simulink model "Inverted_Pendulum_on_a_Cart"  (R2018a)
settings: Solver=VariableStepAuto  StartTime=0.0  StopTime=30  RelTol=1e-3
values from neighbouring files (symbols this model uses):
  g = -9.81    [Matlab_Inverted_Pendulum_on_a_Cart.m]
  l = 2    [Matlab_Inverted_Pendulum_on_a_Cart.m]
  M = 5    [Matlab_Inverted_Pendulum_on_a_Cart.m]
  m = 1    [Matlab_Inverted_Pendulum_on_a_Cart.m]
undefined symbols (not defined in the file or in its folder): magnitude
settings Model: Creator=lucas  LastModifiedBy=root
settings DataIOCC: ReturnWorkspaceOutputs=on
settings SFSimCC: SimUseLocalCustomCode=on
settings RTWCC: RTWUseLocalCustomCode=on

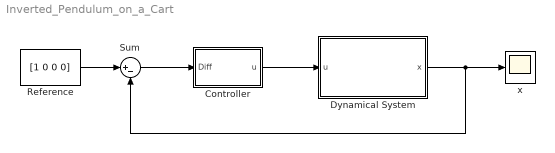
== system Inverted_Pendulum_on_a_Cart ==
  Controller : Subsystem
  Dynamical System : Subsystem
  Reference : Constant  Value=[1 0 0 0]  VectorParams1D=off
  Sum : Sum  Inputs=|+-
  x : Scope
  wires:
  Reference/1 -> Sum/1
  Sum/1 -> Controller/1(Diff)
  Controller/1(u) -> Dynamical System/1(u)
  Dynamical System/1(x) -> x/1, Sum/2

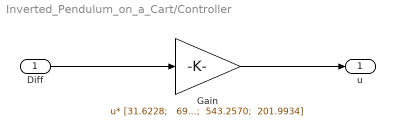
== system Inverted_Pendulum_on_a_Cart/Controller ==
  Diff : Inport
  Gain : Gain  Gain="[31.6228;   69.3926;  543.2570;  201.9934]"  Multiplication=Matrix(u*K)
  u : Outport
  wires:
  Diff/1 -> Gain/1
  Gain/1 -> u/1

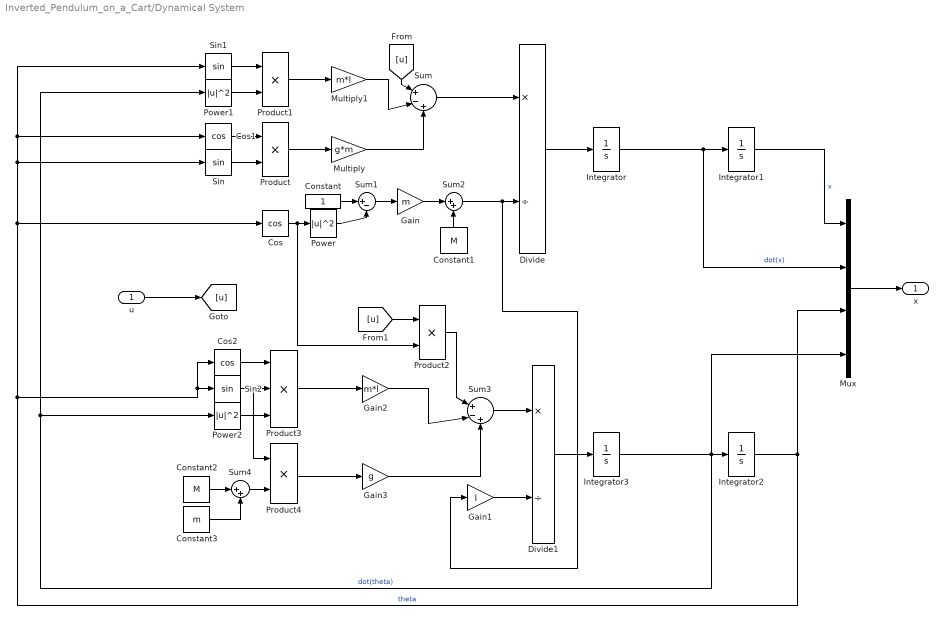
== system Inverted_Pendulum_on_a_Cart/Dynamical System ==
  u : Inport
  Constant : Constant
  Constant1 : Constant  Value=M
  Constant2 : Constant  Value=M
  Constant3 : Constant  Value=m
  Cos : Trigonometry  Operator=cos
  Cos1 : Trigonometry  Operator=cos
  Cos2 : Trigonometry  Operator=cos
  Divide : Product  Inputs=*/
  Divide1 : Product  Inputs=*/
  Gain : Gain  Gain=m
  Gain1 : Gain  Gain=l
  Gain2 : Gain  Gain=m*l
  Gain3 : Gain  Gain=g
  Integrator : Integrator
  Integrator1 : Integrator  InitialCondition=-2
  Integrator2 : Integrator
  Integrator3 : Integrator  InitialCondition=0.7
  Multiply : Gain  Gain=g*m
  Multiply1 : Gain  Gain=m*l
  Mux : Mux
  Power : Math  Operator=magnitude^2  SaturateOnIntegerOverflow=on
  Power1 : Math  Operator=magnitude^2  SaturateOnIntegerOverflow=on
  Power2 : Math  Operator=magnitude^2  SaturateOnIntegerOverflow=on
  Product{,1..2,4} (4 alike) : Product
  Product3 : Product  Inputs=3
  Sin : Trigonometry
  Sin1 : Trigonometry
  Sin2 : Trigonometry
  Sum : Sum  Inputs=|+-+
  Sum1 : Sum  Inputs=|+-
  Sum2 : Sum  Inputs=|++
  Sum3 : Sum  Inputs=|+-+
  Sum4 : Sum  Inputs=|++
  x : Outport
  wires:
  Integrator/1 -> Mux/2, Integrator1/1  "dot(x)"
  Integrator1/1 -> Mux/1  "x"
  Integrator2/1 -> Mux/3, Sin1/1, Cos1/1, Sin/1, Cos/1, Cos2/1, Sin2/1  "theta"
  Divide/1 -> Integrator/1
  Sum/1 -> Divide/1
  Cos/1 -> Product2/2, Power/1
  Constant/1 -> Sum1/1
  Power/1 -> Sum1/2
  Sum1/1 -> Gain/1
  Gain/1 -> Sum2/1
  Constant1/1 -> Sum2/2
  Sum2/1 -> Gain1/1, Divide/2
  Integrator3/1 -> Mux/4, Power2/1, Power1/1, Integrator2/1  "dot(theta)"
  Cos1/1 -> Product/1
  Sin/1 -> Product/2
  Product/1 -> Multiply/1
  Multiply/1 -> Sum/3
  Multiply1/1 -> Sum/2
  Product1/1 -> Multiply1/1
  Power1/1 -> Product1/2
  Sin1/1 -> Product1/1
  Divide1/1 -> Integrator3/1
  Gain1/1 -> Divide1/2
  Sum3/1 -> Divide1/1
  u/1 -> [u]
  [u] -> Sum/1
  [u] -> Product2/1
  Product2/1 -> Sum3/1
  Gain2/1 -> Sum3/2
  Product3/1 -> Gain2/1
  Power2/1 -> Product3/3
  Sin2/1 -> Product4/1, Product3/2
  Cos2/1 -> Product3/1
  Mux/1 -> x/1
  Gain3/1 -> Sum3/3
  Product4/1 -> Gain3/1
  Constant2/1 -> Sum4/1
  Sum4/1 -> Product4/2
  Constant3/1 -> Sum4/2
